simulink model "PendulumDynamics"  (R2022a)
settings: Solver=VariableStepAuto  StartTime=0.0  StopTime=inf  RelTol=1e-3
values from neighbouring files (symbols this model uses):
  A = zeros(2)    [InvertedPendulum.m]    (also in RunSingleJointedArm.m = [0, 1)
  B = -eye(2)/Ts    [InvertedPendulum.m]    (also in RunSingleJointedArm.m = [0)
  C = [0 0; 1 0; 0 0; 0 1]    [InvertedPendulum.m]    (also in RunSingleJointedArm.m = eye(2))
  D = [1 0; 1/Ts 0; 0 1; 0 1/Ts]    [InvertedPendulum.m]    (also in RunSingleJointedArm.m = [0; 0])
  K = [0 -18 -166.5 -15.2]    [InvertedPendulum.m]    (also in RunSingleJointedArm.m = place(A, B, poles))
  l = 0.61 / 2    (= 0.305)    [InvertedPendulum.m]    (also in RunSingleJointedArm.m = 1.2192)
  m = 0.21    [InvertedPendulum.m]    (also in RunSingleJointedArm.m = 2.2675)
  Mcart = 0.455    [InvertedPendulum.m]
  Ts = 0.02    [InvertedPendulum.m]
settings Model: Creator=woz4t  LastModifiedBy=woz4t

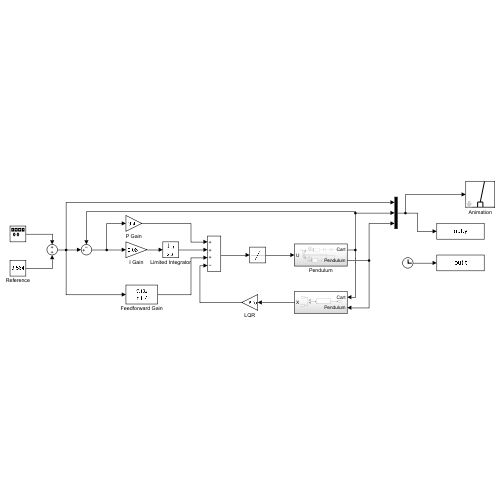
[thumbnail: Simulink's stored preview of the top-level diagram]
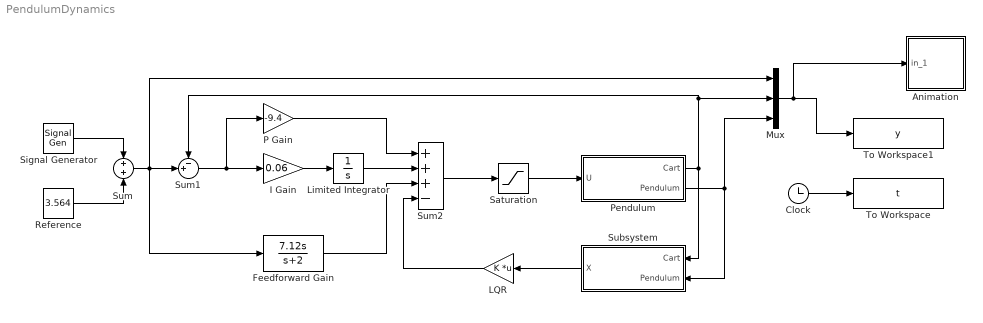
== system PendulumDynamics ==
  Animation : Subsystem  mask(Pendulum plot){RefBlock=Reference}
      mask prompts: RefBlock "DC reference signal block name:"
      mask help: Pendulum plot
      mask Help: Pendulum animation function using Handle graphics.
      mask Display: plot([-10 10],[0 0],[-2 -2 2 2],[0 1 1 0],[0 3],[1 5])
  Clock : Clock
  Feedforward Gain : TransferFcn  Numerator=[7.12 0]  Denominator=[1 2]
  I Gain : Gain  Gain=0.06
  LQR : Gain  Gain=K  Multiplication=Matrix(K*u)
  Limited Integrator : Integrator  LimitOutput=on  UpperSaturationLimit=5  LowerSaturationLimit=-5
  Mux : Mux  Inputs=3
  P Gain : Gain  Gain=-9.4
  Pendulum : Subsystem
  Reference : Constant  Value=3.564
  Saturation : Saturate  UpperLimit=10  LowerLimit=-10
  Signal Generator : SignalGenerator  WaveForm=square  Frequency=0.4  Units=rad/sec
  Subsystem : Subsystem
  Sum : Sum
  Sum1 : Sum  Inputs=-+|
  Sum2 : Sum  Inputs=+++-
  To Workspace : ToWorkspace  VariableName=t  SaveFormat=Timeseries  SampleTime=-1
  To Workspace1 : ToWorkspace  VariableName=y  SaveFormat=Timeseries  SampleTime=-1
  wires:
  Reference/1 -> Sum/2
  Signal Generator/1 -> Sum/1
  Sum/1 -> Mux/1, Feedforward Gain/1, Sum1/2
  Sum1/1 -> P Gain/1, I Gain/1
  I Gain/1 -> Limited Integrator/1
  Limited Integrator/1 -> Sum2/2
  P Gain/1 -> Sum2/1
  Feedforward Gain/1 -> Sum2/3
  Sum2/1 -> Saturation/1
  Saturation/1 -> Pendulum/1(U)
  Pendulum/1(Cart) -> Subsystem/1(Cart), Sum1/1, Mux/2
  Pendulum/2(Pendulum) -> Subsystem/2(Pendulum), Mux/3
  Clock/1 -> To Workspace/1
  Mux/1 -> Animation/1(in_1), To Workspace1/1
  Subsystem/1(X) -> LQR/1
  LQR/1 -> Sum2/4

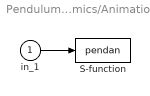
== system PendulumDynamics/Animation ==
  in_1 : Inport
  S-function : S-Function  FunctionName=pendan  Parameters=RefBlock  SFunctionDeploymentMode=off  EnableBusSupport=off
      settings: DeleteFcn=pendan([],[],[],'DeleteBlock');
  wires:
  in_1/1 -> S-function/1

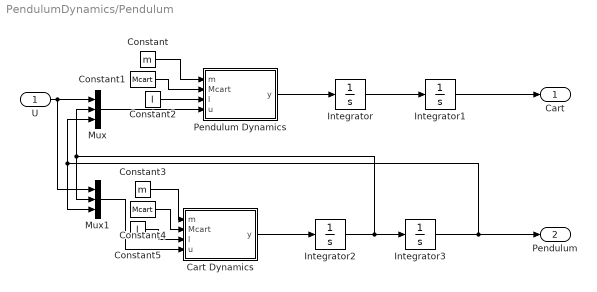
== system PendulumDynamics/Pendulum ==
  U : Inport
  Cart Dynamics : MATLAB Function  TreatAsAtomicUnit=on
  Constant : Constant  Value=m
  Constant1 : Constant  Value=Mcart
  Constant2 : Constant  Value=l
  Constant3 : Constant  Value=m
  Constant4 : Constant  Value=Mcart
  Constant5 : Constant  Value=l
  Integrator{,1..3} (4 alike) : Integrator
  Mux : Mux  Inputs=3
  Mux1 : Mux  Inputs=3
  Pendulum Dynamics : MATLAB Function  TreatAsAtomicUnit=on
  Cart : Outport
  Pendulum : Outport  Port=2
  wires:
  U/1 -> Mux1/1, Mux/1
  Mux/1 -> Pendulum Dynamics/4(u)
  Mux1/1 -> Cart Dynamics/4(u)
  Pendulum Dynamics/1(y) -> Integrator/1
  Integrator/1 -> Integrator1/1
  Integrator1/1 -> Cart/1
  Integrator2/1 -> Mux/2, Mux1/2, Integrator3/1
  Cart Dynamics/1(y) -> Integrator2/1
  Integrator3/1 -> Mux/3, Mux1/3, Pendulum/1
  Constant/1 -> Pendulum Dynamics/1(m)
  Constant2/1 -> Pendulum Dynamics/3(l)
  Constant1/1 -> Pendulum Dynamics/2(Mcart)
  Constant3/1 -> Cart Dynamics/1(m)
  Constant5/1 -> Cart Dynamics/3(l)
  Constant4/1 -> Cart Dynamics/2(Mcart)

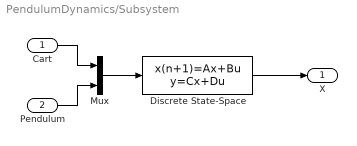
== system PendulumDynamics/Subsystem ==
  Cart : Inport
  Pendulum : Inport  Port=2
  Discrete State-Space : DiscreteStateSpace  A=A  B=B  C=C  D=D  SampleTime=Ts
  Mux : Mux  Inputs=2
  X : Outport
  wires:
  Cart/1 -> Mux/1
  Pendulum/1 -> Mux/2
  Mux/1 -> Discrete State-Space/1
  Discrete State-Space/1 -> X/1

== matlab function PendulumDynamics/Pendulum/Cart Dynamics ==
  data: m input; Mcart input; l input; u input; y output
function y = CartDynamics(m, Mcart, l, u)

g = 9.81;
y = (-u(1)*cos(u(3))/m + (Mcart+m)*g*sin(u(3))/m - l*power(u(2),2)*sin(u(3))*cos(u(3)))/(l*(Mcart/m + power(sin(u(3)),2)));
end

== matlab function PendulumDynamics/Pendulum/Pendulum Dynamics ==
  data: m input; Mcart input; l input; u input; y output
function y = PendulumDynamics(m, Mcart, l, u)

g = 9.81;
y = (u(1)/m - g*sin(u(3))*cos(u(3)) + l*power(u(2),2)*sin(u(3)))/(Mcart/m + power(sin(u(3)),2));

end
